simulink model "ques8_stateflow"  (R2020b)
settings: Solver=VariableStepAuto  StartTime=0.0  StopTime=10.0  RelTol=1e-3
settings Model: Creator=sneha  LastModifiedBy=sneha

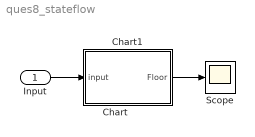
== system ques8_stateflow ==
  Input : Inport
  Chart : Stateflow chart  TreatAsAtomicUnit=on
  Chart1 : Stateflow chart  TreatAsAtomicUnit=on
  Scope : Scope
  wires:
  Chart1/1(Floor) -> Scope/1
  Input/1 -> Chart1/1(input)

== stateflow chart ques8_stateflow/Chart1 ==
  state ModelLift [parallel]
    settings: executionOrder=1
    state LiftLocation
      state FloorFive
        entry:
        Floor =5;
        opendoor = goto - Floor +1
      state FloorFour
        entry:
        Floor = 4;
        opendoor = goto - Floor +1
      state FloorThree
        entry:
        Floor = 3;
        opendoor = goto - Floor +1
      state FloorTwo
        entry:
        Floor = 2;
        opendoor = goto - Floor +1
      state FloorOne
        entry:
        Floor = 1;
        opendoor = goto - Floor +1
        during:
        wait = 1+1;
      (default) -> FloorFive
      FloorFive -> FloorFive [order 2] : [goto==0]
      FloorFive -> FloorFour [order 1] : [goto<Floor]{doorOpened=0}
      FloorFour -> FloorFive [order 2] : [goto>Floor]{doorOpened=0}
      FloorFour -> FloorFour [order 3] : [goto==0]
      FloorFour -> FloorThree [order 1] : [goto<Floor]{doorOpened=0}
      FloorThree -> FloorFour [order 2] : [goto>Floor]{doorOpened=0}
      FloorThree -> FloorThree [order 3] : [goto==0]
      FloorThree -> FloorTwo [order 1] : [goto<Floor]{doorOpened=0}
      FloorTwo -> FloorThree [order 2] : [goto>Floor]{doorOpened=0}
      FloorTwo -> FloorTwo [order 3] : [goto==0]
      FloorTwo -> FloorOne [order 1] : [goto<Floor]{doorOpened=0}
      FloorOne -> FloorTwo [order 1] : [goto>Floor]{doorOpened=0}
      FloorOne -> FloorOne [order 2] : [goto==0]
    state DoorState
      state OpenDoor
        exit:
      state CloseDoor
        %goto = queue(1);
      (default) -> OpenDoor
      OpenDoor -> (junction 10)
      (junction 10) -> CloseDoor : after(2,sec)
    (default) -> LiftLocation
    LiftLocation -> (junction 60) : [opendoor==1]
    (junction 60) -> (junction 61) : [doorOpened==0]
    (junction 61) -> DoorState : {floorReached=1}
    CloseDoor -> LiftLocation : after(1,sec){doorOpened=1}
  state FloorInQueue [parallel]
    settings: executionOrder=2
    state InitializeQueue
      entry:
      n = 0;
      temp = input;
    state Checker
      en:
      checkVals(input,queue(i));
      i = i+1;
    state AddQueue
      entry:
      n=n+1;
      queue(n) = temp;
      goto = queue(1);
      addVal =0;
    state IDLE
      en:
      i = 1
      addVal = 1;
      temp = input;
    state RemoveFirst
      entry:
      queue(i) = queue(i+1);
      i = i+1;
      floorReached = 0;
    (default) -> InitializeQueue
    Checker -> Checker [order 2] : [queue(i)~=0]
    InitializeQueue -> AddQueue : [input>0]{temp=input}
    IDLE -> Checker [order 1] : [temp~=input]
    Checker -> (junction 88) [order 1] : [addVal==1]
    (junction 88) -> AddQueue : {temp=input}
    AddQueue -> IDLE
    RemoveFirst -> RemoveFirst [order 1] : [queue(i)~=0]
    IDLE -> RemoveFirst [order 2] : [floorReached==1]
    (junction 85) -> IDLE : {goto=queue(1)}
    RemoveFirst -> (junction 85) [order 2] : {n=n-1}
  state checkVals(data1,data2) [function]
    (default) -> (junction 105)
    (junction 105) -> (junction 103) [order 1] : [data1 == data2]
    (junction 105) -> (junction 108) [order 2]
    (junction 103) -> (junction 106) : {addVal = 0;}
    (junction 106) -> (junction 108)
    (junction 108) -> (junction 104)
  data: data1 function_input; data2 function_input; goto local =1; Floor output; wait local; opendoor local; doorOpened local; floorReached local =0; addVal local =0; temp local =0; i local =1; queue local =[0 0 0 0 0 0 0 0 0 0]; n local; input input

== stateflow chart ques8_stateflow/Chart ==
